simulink subsystem "Estimation_old"  (R2022a)
settings: Solver=VariableStepAuto  StartTime=0.0  StopTime=10.0  RelTol=1e-3
undefined symbols (not defined in the file): vy0, yaw_rate0
settings Model: Creator=jutri  LastModifiedBy=Usuario
settings ModelReferenceCC: EnableRefExpFcnMdlSchedulingChecks=off
settings RTWCC: Description=Generic Real-Time Target  GPUComputeCapability=5.0

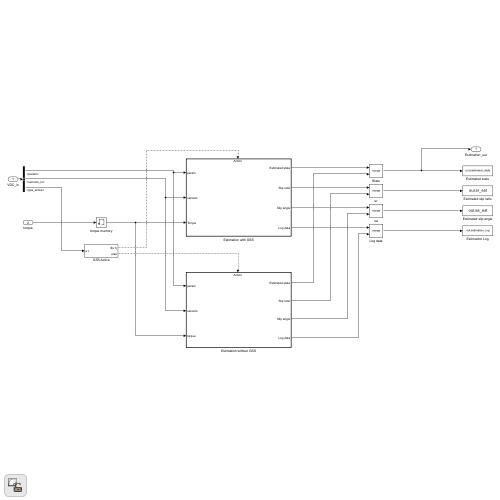
[thumbnail: Simulink's stored preview of the top-level diagram]
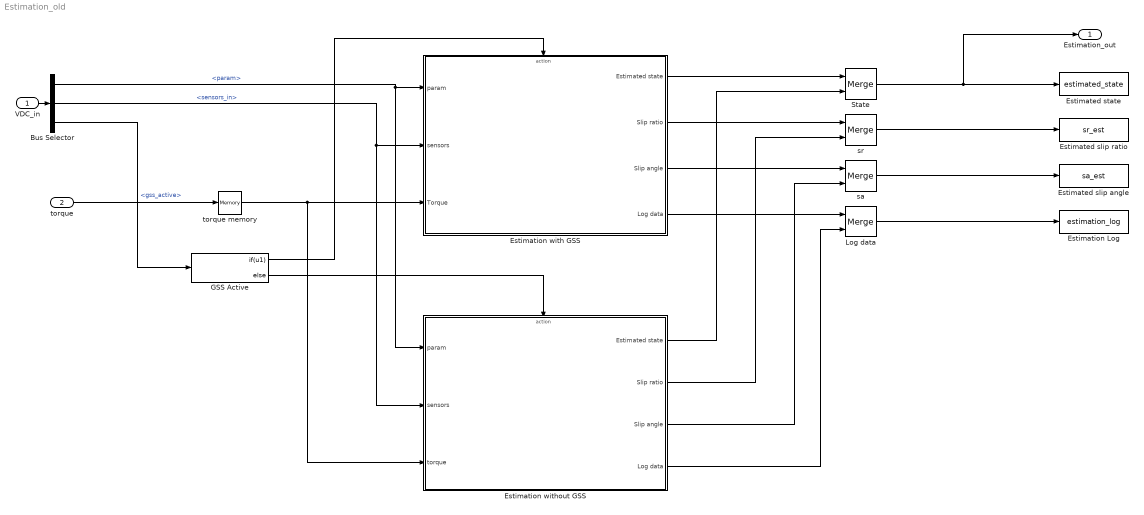
== system Estimation_old ==
  VDC_in : Inport
  torque : Inport  Port=2
  Bus Selector : BusSelector  OutputSignals=param,sensors_in,param.gss_active
  Estimated slip angle : ToWorkspace  VariableName=sa_est  SaveFormat=Timeseries  SampleTime=-1
  Estimated slip ratio : ToWorkspace  VariableName=sr_est  SaveFormat=Timeseries  SampleTime=-1
  Estimated state : ToWorkspace  VariableName=estimated_state  SaveFormat=Timeseries  SampleTime=-1
      settings: Decimation=3
  Estimation Log : ToWorkspace  VariableName=estimation_log  SaveFormat=Timeseries  SampleTime=-1
  Estimation with GSS : Subsystem  TreatAsAtomicUnit=on
  Estimation without GSS : Subsystem  TreatAsAtomicUnit=on
  GSS Active : If  IfExpression=u1
  Log data : Merge
  State : Merge
  sa : Merge
  sr : Merge
  torque memory : Memory  InitialCondition=zeros(4,1)
  Estimation_out : Outport
  wires:
  VDC_in/1 -> Bus Selector/1
  Bus Selector/3 -> GSS Active/1  "<gss_active>"
  Bus Selector/1 -> Estimation without GSS/1(param), Estimation with GSS/1(param)  "<param>"
  Bus Selector/2 -> Estimation without GSS/2(sensors), Estimation with GSS/2(sensors)  "<sensors_in>"
  torque/1 -> torque memory/1
  State/1 -> Estimation_out/1, Estimated state/1
  sr/1 -> Estimated slip ratio/1
  sa/1 -> Estimated slip angle/1
  GSS Active/2 -> Estimation without GSS/Action
  GSS Active/1 -> Estimation with GSS/Action
  Estimation with GSS/1(Estimated state) -> State/1
  Estimation with GSS/2(Slip ratio) -> sr/1
  Estimation with GSS/3(Slip angle) -> sa/1
  Estimation without GSS/1(Estimated state) -> State/2
  Estimation without GSS/2(Slip ratio) -> sr/2
  Estimation without GSS/3(Slip angle) -> sa/2
  torque memory/1 -> Estimation without GSS/3(torque), Estimation with GSS/3(Torque)
  Estimation with GSS/4(Log data) -> Log data/1
  Estimation without GSS/4(Log data) -> Log data/2
  Log data/1 -> Estimation Log/1

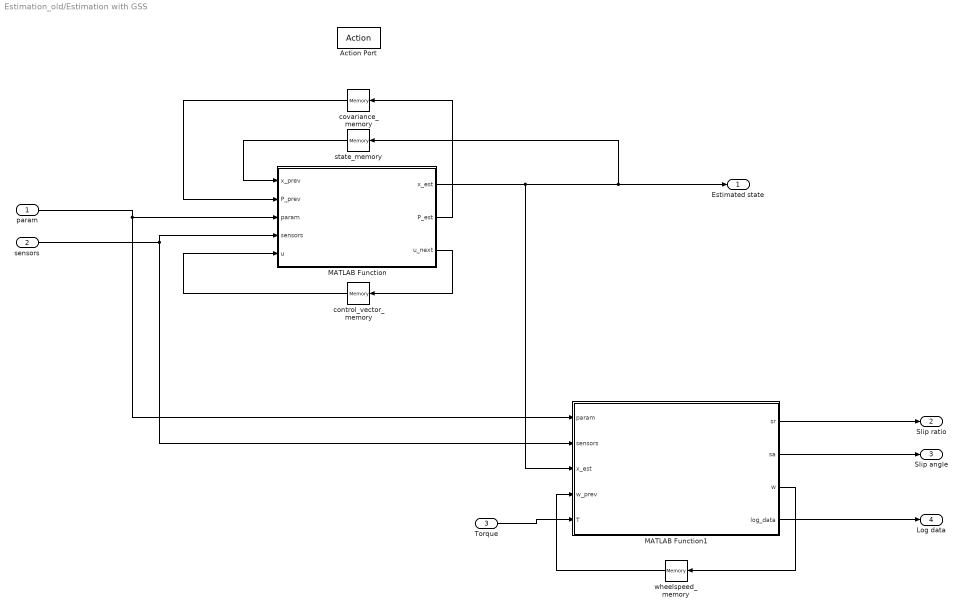
== system Estimation_old/Estimation with GSS ==
  param : Inport
  sensors : Inport  Port=2
  Torque : Inport  Port=3
  Action Port : ActionPort
  MATLAB Function : MATLAB Function  TreatAsAtomicUnit=on
  MATLAB Function1 : MATLAB Function  TreatAsAtomicUnit=on
  control_vector_memory : Memory  InitialCondition=[0; 0]
  covariance_memory : Memory  InitialCondition=diag(0.1*ones(3,1))
  state_memory : Memory  InitialCondition=[0; vy0; yaw_rate0]
  wheelspeed_memory : Memory  InitialCondition=zeros(4,1)
  Estimated state : Outport
  Slip ratio : Outport  Port=2
  Slip angle : Outport  Port=3
  Log data : Outport  Port=4
  wires:
  state_memory/1 -> MATLAB Function/1(x_prev)
  MATLAB Function/1(x_est) -> state_memory/1, Estimated state/1, MATLAB Function1/3(x_est)
  MATLAB Function/2(P_est) -> covariance_memory/1
  control_vector_memory/1 -> MATLAB Function/5(u)
  sensors/1 -> MATLAB Function/4(sensors), MATLAB Function1/2(sensors)
  MATLAB Function/3(u_next) -> control_vector_memory/1
  covariance_memory/1 -> MATLAB Function/2(P_prev)
  MATLAB Function1/1(sr) -> Slip ratio/1
  param/1 -> MATLAB Function/3(param), MATLAB Function1/1(param)
  MATLAB Function1/2(sa) -> Slip angle/1
  MATLAB Function1/3(w) -> wheelspeed_memory/1
  wheelspeed_memory/1 -> MATLAB Function1/4(w_prev)
  Torque/1 -> MATLAB Function1/5(T)
  MATLAB Function1/4(log_data) -> Log data/1

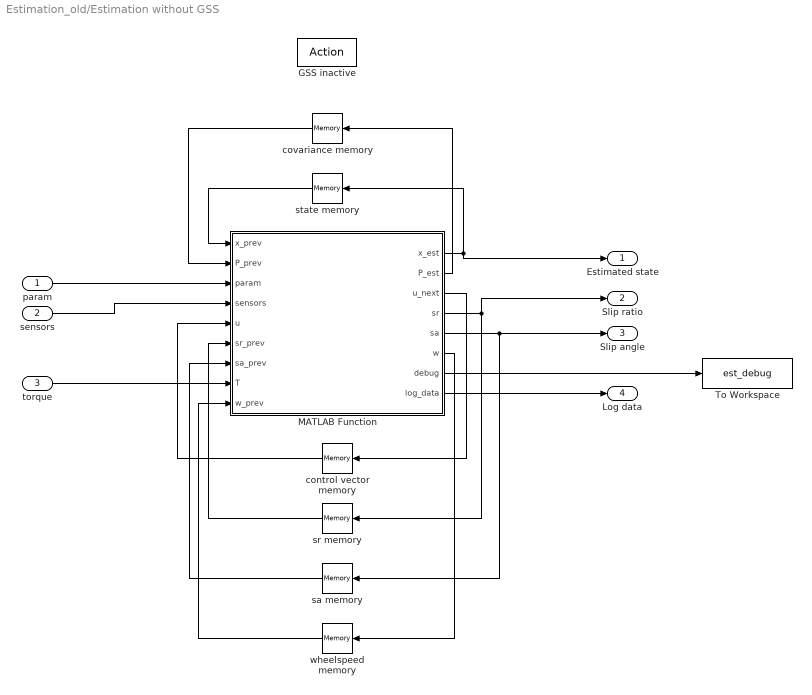
== system Estimation_old/Estimation without GSS ==
  param : Inport
  sensors : Inport  Port=2
  torque : Inport  Port=3
  GSS inactive : ActionPort
  MATLAB Function : MATLAB Function  TreatAsAtomicUnit=on
  To Workspace : ToWorkspace  VariableName=est_debug  SaveFormat=Timeseries  SampleTime=-1
  control vector memory : Memory  InitialCondition=[0;0]
  covariance memory : Memory  InitialCondition=diag(0.1*ones(3,1))
  sa memory : Memory  InitialCondition=zeros(4,1)
  sr memory : Memory  InitialCondition=zeros(4,1)
  state memory : Memory  InitialCondition=[0; vy0; yaw_rate0]
  wheelspeed memory : Memory  InitialCondition=zeros(4,1)
  Estimated state : Outport
  Slip ratio : Outport  Port=2
  Slip angle : Outport  Port=3
  Log data : Outport  Port=4
  wires:
  MATLAB Function/7(debug) -> To Workspace/1
  wheelspeed memory/1 -> MATLAB Function/9(w_prev)
  MATLAB Function/6(w) -> wheelspeed memory/1
  torque/1 -> MATLAB Function/8(T)
  sa memory/1 -> MATLAB Function/7(sa_prev)
  MATLAB Function/5(sa) -> sa memory/1, Slip angle/1
  sr memory/1 -> MATLAB Function/6(sr_prev)
  MATLAB Function/4(sr) -> Slip ratio/1, sr memory/1
  control vector memory/1 -> MATLAB Function/5(u)
  MATLAB Function/3(u_next) -> control vector memory/1
  sensors/1 -> MATLAB Function/4(sensors)
  param/1 -> MATLAB Function/3(param)
  covariance memory/1 -> MATLAB Function/2(P_prev)
  MATLAB Function/2(P_est) -> covariance memory/1
  state memory/1 -> MATLAB Function/1(x_prev)
  MATLAB Function/1(x_est) -> state memory/1, Estimated state/1
  MATLAB Function/8(log_data) -> Log data/1

== matlab function Estimation_old/Estimation with GSS/MATLAB Function ==
  data: x_prev input; P_prev input; param input; sensors input; x_est output; P_est output; u input; u_next output
function [x_est, P_est, u_next] = state_estimation(x_prev, P_prev, param, sensors, u)
% State vector: x = [vx; vy; wz]
    % vx    - Longitudinal velocity
    % vy    - Lateral velocity
    % wz    - Yaw rate

% Input:
%  x_prev   - Previously estimated state.
%  P_prev   - Previously estimaded state covariance matrix.
%  param    - Car's parameters, detailed in vdc-ART25/Parameters.
%  sensors  - Sensor data, stored in struct as follows:
%       IMU
%           r    - Yaw rate [rad/s]
%           ax   - Longitudinal acceleration [m/s^2]
%           ay   - Lateral acceleration [m/s^2]
%       encoder
%           wFL  - Wheelspeed FL [rad/s]
%           wFR  - Wheelspeed FR [rad/s]
%           wRL  - Wheelspeed RL [rad/s]
%           wRR  - Wheelspeed RR [rad/s]
%       ext
%           steering  - steering angle [rad]
%       gss
%           vx   - Longitudinal velocity [m/s]
%           vy   - Lateral velocity [m/s]

%  u        - Control vector u = [ax_prev; delta_prev]   

% Output:
% estimated_state       - Estimated state.
% estimated_covariance  - Estimated state covariance matrix.
% u_next                - Control vector for next iteration

dt = param.TimeStep;
nx = length(x_prev);

%% Velocity estimator (Simple KF)
% Tire cornering stiffness
cf = 26*1e3;
cr = 24*1e3;

% Process covariance matrix
Q = diag([0.025, 0.005, 0.01]);

% Measurement covariance matrix
R = diag([0.01, 0.005, 0.002]);

% Kalman model matrices
% Transition matrix
vx_prev = x_prev(1);

if(vx_prev < param.vx_threshold)
    A = eye(nx);
else
    A = eye(nx) + dt * [0, 0, 0;
                    0, -(cf + cr) / (param.mass * vx_prev), ...
                        (param.lr * cr - param.lf * cf) / (param.mass * vx_prev) - vx_prev;
                    0, (param.lr * cr - param.lf * cf) / (param.Iz * vx_prev), ...
                        -(param.lf^2 * cf + param.lr^2 * cr) / (param.Iz * vx_prev)];   
end

% Control matrix
B = [1, 0;
     0, cf / param.mass;
     0, cf * param.lf / param.Iz];

% Observation matrix
H = eye(nx);

%% PREDICTION STAGE
% State prediction
x_pred = A * x_prev + dt * B * u;
P_pred = A * P_prev * A' + Q;

% Measurement prediciton
z = [sensors.gss.vx; sensors.gss.vy; sensors.IMU.r];
z_pred = H * x_pred;

% Kalman gain
K = P_pred * H' / (H * P_pred * H' + R);

%% UPDATE STAGE
% State estimation
x_est = x_pred + K * (z - z_pred);
P_est = (eye(nx) - K * H) * P_pred;

% Control vector update
delta = sensors.ext.steering;
u_next = [sensors.IMU.ax; delta];

== matlab function Estimation_old/Estimation with GSS/MATLAB Function1 ==
  data: param input; sr output; sensors input; x_est input; sa output; w_prev input; T input; w output; log_data output
function [sr, sa, w, log_data] = slip_estimation(param, sensors, x_est, w_prev, T)
tf = param.trackwidthF;
tr = param.trackwidthR;
lf = param.lf;
    lr = param.lr;
r = param.rdyn;
dt = param.TimeStep;

delta_ext = sensors.ext.steering;
delta =  calculate_steering(delta_ext, param);

% Combine direct formula and TMEasy inverse
Tr = [cos(delta(1)),  sin(delta(1)), -0.5*tf*cos(delta(1)) + lf*sin(delta(1));
    cos(delta(2)),   sin(delta(2)), 0.5*tf*cos(delta(2)) + lf*sin(delta(2));
    1,            0,          -0.5*tr;
    1,            0,          0.5*tr;
    -sin(delta(1)),  cos(delta(1)), lf*cos(delta(1)) + 0.5*tf*sin(delta(1));
    -sin(delta(2)),  cos(delta(2)), lf*cos(delta(2)) - 0.5*tf*sin(delta(2));
    0,            1,          -lr;
    0,            1,          -lr];


v_w = Tr * x_est;
v_wx = v_w(1:4);
v_wy = v_w(5:8);
w = [sensors.encoder.wFL; sensors.encoder.wFR; sensors.encoder.wRL; sensors.encoder.wRR];


sr = r * w ./ v_wx - 1;
for i=1:4
    if(v_wx(i) < 1)
        sr(i) = r * w(i) - v_wx(i);
    end
end

sa = atan2(v_wy, v_wx);

%% Generate estimation log
v = sqrt(x_est(1)^2 + x_est(2)^2);
alpha = (w - w_prev)/dt;
[F_wx, F_wy, F_wz] = estimate_tire_forces(sensors,param,v,T,alpha);

sensor_vec = [sensors.IMU.r; sensors.IMU.ax; sensors.IMU.ay; sensors.encoder.wFL; sensors.encoder.wFR; sensors.encoder.wRL; sensors.encoder.wRR; ...
    sensors.ext.steering; sensors.gss.vx; sensors.gss.vy];
phi = atan2(F_wy, F_wx);
log_data = [sensor_vec; T; x_est; sr; sa; F_wz; phi];

== matlab function Estimation_old/Estimation without GSS/MATLAB Function ==
  data: x_prev input; P_prev input; param input; sensors input; u input; sr_prev input; sa_prev input; x_est output; P_est output; u_next output; sr output; sa output; T input; w_prev input; w output; debug output; log_data output
function [x_est, P_est, u_next, sr, sa, w, debug, log_data] = state_estimation(x_prev, P_prev, param, sensors, u, sr_prev, sa_prev, T, w_prev)
% State vector: x = [vx; vy; wz]
    % vx    - Longitudinal velocity
    % vy    - Lateral velocity
    % wz    - Yaw rate

% Input:
%  x_prev   - Previously estimated state.
%  P_prev   - Previously estimaded state covariance matrix.
%  param    - Car's parameters, detailed in vdc-ART25/Parameters.
%  sensors  - Sensor data, stored in struct as follows:
%       IMU
%           r    - Yaw rate [rad/s]
%           ax   - Longitudinal acceleration [m/s^2]
%           ay   - Lateral acceleration [m/s^2]
%       encoder
%           wFL  - Wheelspeed FL [rad/s]
%           wFR  - Wheelspeed FR [rad/s]
%           wRL  - Wheelspeed RL [rad/s]
%           wRR  - Wheelspeed RR [rad/s]
%       ext
%           steering  - steering angle [rad]
%  u        - Control vector u = [ax_prev; delta_prev]   

% Output:
% x_est       - Estimated state.
% P_est       - Estimated state covariance matrix.
% u_next      - Control vector for next iteration

dt = param.TimeStep;
nx = length(x_prev);

%% Tire inverse model
v_prev = sqrt(x_prev(1)^2 + x_prev(2)^2);
w = [sensors.encoder.wFL; sensors.encoder.wFR; sensors.encoder.wRL; sensors.encoder.wRR];
alpha = (w - w_prev)/dt;

[F_wx, F_wy, F_wz] = estimate_tire_forces(sensors, param, v_prev, T, alpha);
[sr_TME, sa] = TMEasy_inverse_model(F_wx, F_wy, F_wz, sr_prev, sa_prev,true);

%% Slip ratio / angle definition
delta_ext = sensors.ext.steering;
delta = calculate_steering(delta_ext, param);

v_wx = (w*param.rdyn) ./ (sr_TME + 1);
v_wy = tan(sa) .* v_wx; 

%% Velocity estimator (Simple KF)
% Tire cornering stiffness
cf = 26*1e3;
cr = 24*1e3;

% Process covariance matrix
Q = diag([0.025, 0.01, 0.01]);

% Measurement covariance matrix
R = diag([0.015*ones(1,4), 0.05*ones(1,2), 0.025*ones(1,2), 0.002]);

% Kalman model matrices
% Transition matrix
vx_prev = x_prev(1);

if(vx_prev < param.vx_threshold)
    A = eye(nx);
else
    A = eye(nx) + dt * [0, 0, 0;
                    0, -(cf + cr) / (param.mass * vx_prev), ...
                        (param.lr * cr - param.lf * cf) / (param.mass * vx_prev) - vx_prev;
                    0, (param.lr * cr - param.lf * cf) / (param.Iz * vx_prev), ...
                        -(param.lf^2 * cf + param.lr^2 * cr) / (param.Iz * vx_prev)];   
end    

% Control matrix
B = [1, 0;
     0, cf / param.mass;
     0, cf * param.lf / param.Iz];

% Observation matrix
H = [cos(delta(1)),  sin(delta(1)), -0.5*param.trackwidthF*cos(delta(1)) + param.lf*sin(delta(1));
    cos(delta(2)),   sin(delta(2)), 0.5*param.trackwidthF*cos(delta(2)) + param.lf*sin(delta(2));
    1,            0,          -0.5*param.trackwidthR;
    1,            0,          0.5*param.trackwidthR;
    -sin(delta(1)),  cos(delta(1)), param.lf*cos(delta(1)) + 0.5*param.trackwidthF*sin(delta(1));
    -sin(delta(2)),  cos(delta(2)), param.lf*cos(delta(2)) - 0.5*param.trackwidthF*sin(delta(2));
    0,            1,          -param.lr;
    0,            1,          -param.lr;
    0,            0,          1];

%% PREDICTION STAGE
% State prediction
x_pred = A * x_prev + dt * B * u;
P_pred = A * P_prev * A' + Q;

% Measurement prediciton
z = [v_wx; v_wy; sensors.IMU.r];
z_pred = H * x_pred;

% Kalman gain
K = P_pred * H' / (H * P_pred * H' + R);

%% UPDATE STAGE
% State estimation
x_est = x_pred + K * (z - z_pred);
P_est = (eye(nx) - K * H) * P_pred;


% x_est = [0.5*((z(3)+0.5*param.trackwidthR*z(9)) + (z(4)-0.5*param.trackwidthR*z(9)));
%         0.5*((z(7)+param.lr*z(9)) + (z(8)+param.lr*z(9)));
%         z(9)];


% Control vector update
u_next = [sensors.IMU.ax; delta_ext];

debug = [v_wx; v_wy];

%% Correct slip ratio calculation
sr = zeros(4,1);
z_est = H * x_est;
v_wx = z_est(1:4);

for i=1:4
    if(abs(sr_prev(i)) < 0.02)
        sr(i) = sr_TME(i);
    else
        if(v_wx(i) < 1)
            sr(i) = param.rdyn * w(i) - v_wx(i);
        else
            sr(i) = param.rdyn * w(i) ./ v_wx(i) - 1;
        end
    end
end

%% Generate estimation log
sensor_vec = [sensors.IMU.r; sensors.IMU.ax; sensors.IMU.ay; sensors.encoder.wFL; sensors.encoder.wFR; sensors.encoder.wRL; sensors.encoder.wRR; ...
    sensors.ext.steering; sensors.gss.vx; sensors.gss.vy];
phi = atan2(F_wy, F_wx);
log_data = [sensor_vec; T; x_est; sr; sa; F_wz; phi];
